simulink model "first"  (R2022b)
settings: Solver=VariableStepAuto  StartTime=0.0  StopTime=10.0  RelTol=1e-3
libraries: simulink x2
settings Model: Creator=adnzw  LastModifiedBy=adnzw

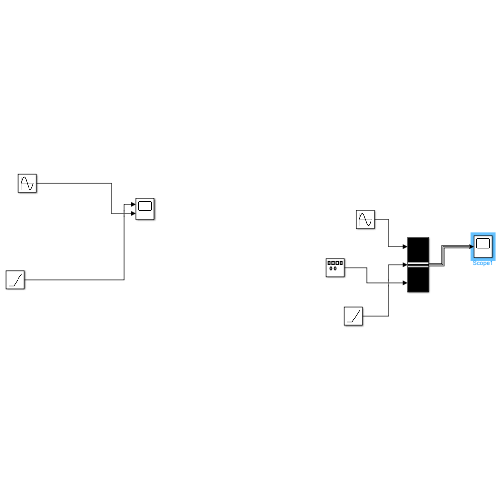
[thumbnail: Simulink's stored preview of the top-level diagram]
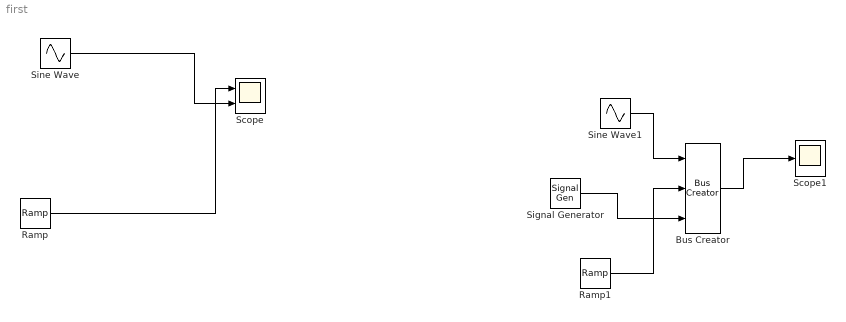
== system first ==
  Bus Creator : BusCreator  Inputs=3
  Ramp : simulink/Sources/Ramp  slope=1  start=0  InitialOutput=0
  Ramp1 : simulink/Sources/Ramp  slope=1  start=0  InitialOutput=0
  Scope : Scope  NumInputPorts=2
  Scope1 : Scope
  Signal Generator : SignalGenerator  WaveForm=square  Units=rad/sec
  Sine Wave : Sin  SampleTime=0
  Sine Wave1 : Sin  SampleTime=0
  wires:
  Ramp/1 -> Scope/1
  Sine Wave/1 -> Scope/2
  Sine Wave1/1 -> Bus Creator/1
  Ramp1/1 -> Bus Creator/2
  Bus Creator/1 -> Scope1/1
  Signal Generator/1 -> Bus Creator/3
